simulink model "k1vistmsy"  (Simulink 8.6)
settings: Solver=ode45  StartTime=0.0  StopTime=10.0  RelTol=1e-3
libraries: VIS_TMS_LIB x3, cdsCDI64 x2, cdsCDO64 x2, cdsIPCx x2, cdsAdcx0 x1, cdsAdcx1 x1, cdsAdcx2 x1, dac x1, simulink x1, cdsParameters x1
settings Model: Creator=controls  LastModifiedBy=controls
settings OptimizationCC: InitFltsAndDblsToZero=on
settings DebuggingCC: FcnCallInpInsideContextMsg=EnableAllAsWarning  AllowSymbolicDim=on  StrictBusMsg=Warning

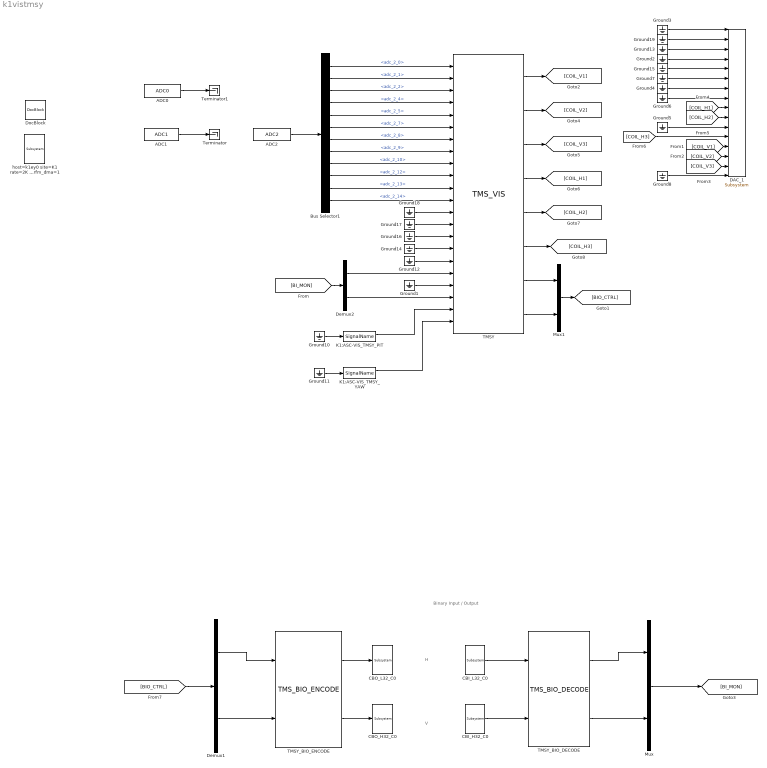
== system k1vistmsy ==
  note: Binary Input / Output
  note: H
  note: V
  ADC0 : cdsAdcx0/ADC0  Tag=cdsAdc  Description=|
      | type-GSC_16AI64SSA
      | card_num=0
      settings: AttributesFormatString=%<Description>\n%<Tag>
  ADC1 : cdsAdcx1/ADC1  Tag=cdsAdc  Description=|
      | type-GSC_16AI64SSA
      | card_num=1
      settings: AttributesFormatString=%<Description>\n%<Tag>
  ADC2 : cdsAdcx2/ADC2  Tag=cdsAdc  Description=|
      | type-GSC_16AI64SSA
      | card_num=2
      settings: AttributesFormatString=%<Description>\n%<Tag>
  Bus Selector1 : BusSelector  Description=ADC Selector  OutputSignals=adc_2_0,adc_2_1,adc_2_2,adc_2_4,adc_2_5,adc_2_7,adc_2_8,adc_2_9,adc_2_10,adc_2_12,adc_2_13,adc_2_14
      settings: AttributesFormatString=%<Description>
  CBI_H32_C0 : cdsCDI64/Subsystem  Tag=cdsCDI64  Description=card_num=1
      settings: AttributesFormatString=%<Tag>\n%<Description>
  CBI_L32_C0 : cdsCDI64/Subsystem  Tag=cdsCDI64  Description=card_num=0
      settings: AttributesFormatString=%<Tag>\n%<Description>
  CBO_H32_C0 : cdsCDO64/Subsystem  Tag=cdsCDO64  Description=card_num=1
      settings: AttributesFormatString=%<Tag>\n%<Description>
  CBO_L32_C0 : cdsCDO64/Subsystem  Tag=cdsCDO64  Description=card_num=0
      settings: AttributesFormatString=%<Tag>\n%<Description>
  DAC_1 : dac/Subsystem  Description=|
      | type=GSC_16AO16,
      | card_num=1
      settings: AttributesFormatString=%<Description>
  Demux1 : Demux  Outputs=2
  Demux2 : Demux  Outputs=2
  DocBlock : simulink/Model-Wide Utilities/DocBlock  DocumentType=Text
  Ground{1..8,10..19} (18 alike) : Ground
  K1:ASC-VIS_TMSY_PIT : cdsIPCx/SignalName  Tag=cdsIPCx_RFM  Description=card=1
      settings: AttributesFormatString=%<Description>\n%<Tag>
  K1:ASC-VIS_TMSY_YAW : cdsIPCx/SignalName  Tag=cdsIPCx_RFM  Description=card=1
      settings: AttributesFormatString=%<Description>\n%<Tag>
  Mux : Mux  Inputs=2
  Mux1 : Mux  Inputs=2
  TMSY : VIS_TMS_LIB/TMS_VIS
  TMSY_BIO_DECODE : VIS_TMS_LIB/TMS_BIO_DECODE
  TMSY_BIO_ENCODE : VIS_TMS_LIB/TMS_BIO_ENCODE
  Terminator : Terminator
  Terminator1 : Terminator
  host=k1ey0 site=K1 rate=2K dcuid=114 specific_cpu=6 adcSlave=1 no_rfm_dma=1 : cdsParameters/Subsystem  Tag=cdsParameters  Description=|
      | Purpose:                                                                                                                                                                                                                                
      |                                                                                                                                                                                                                                         
      | Provide system parameters to the FE code generator to properly configure the generated EPICS names, rep rate of the FE controller, and the Data Acquisition node ID for proper storage of data from this FE controller.                 
      |                                                                                                                                                                                                                                         
      | Useage:                                                                                                                                                                                                                                 
      |                                                                                                                                                                                                                                         
      | The part NAME field is used to identify the FE parameters. It must be of the form:                                                                                                                                                      
      |                                                                                                                                                                                                                                         
      | site=                                                                                                                                                                                                                                   
      | rate=                                                                                                                                                                                                                                   
      | dcuid=                                                                                                                                                                                                                                  
      |                                                                                                                                                                                                                                         
      | Where:                                                                                                                                                                                                                                  
      |                                                                                                                                                                                                                                         
      | site= argument may be H1, H2, L1, M1, G1, either as a single argument or multiple, for example site=H1,H2. These are the only names allowed. These will become the first two characters of all EPICS and signal names (for example G1:).
      |                                                                                                                                                                                                                                         
      | rate= may be 2K, 16K, 32K, or 64K                                                                                                                                                                                                       
      |                                                                                                                                                                                                                                         
      | dcuid= is site specific ie it must be unique at each site.
      settings: AttributesFormatString=%<Tag>
  wires:
  Bus Selector1/10 -> TMSY/10  "<adc_2_12>"
  Bus Selector1/11 -> TMSY/11  "<adc_2_13>"
  Bus Selector1/12 -> TMSY/12  "<adc_2_14>"
  TMSY_BIO_ENCODE/1 -> CBO_L32_C0/1
  CBI_L32_C0/1 -> TMSY_BIO_DECODE/1
  TMSY_BIO_DECODE/2 -> Mux/2
  TMSY_BIO_DECODE/1 -> Mux/1
  Mux/1 -> [BI_MON]
  [BIO_CTRL] -> Demux1/1
  TMSY_BIO_ENCODE/2 -> CBO_H32_C0/1
  Demux1/1 -> TMSY_BIO_ENCODE/1
  Demux1/2 -> TMSY_BIO_ENCODE/2
  CBI_H32_C0/1 -> TMSY_BIO_DECODE/2
  [BI_MON] -> Demux2/1
  TMSY/7 -> Mux1/1
  TMSY/8 -> Mux1/2
  Mux1/1 -> [BIO_CTRL]
  Demux2/1 -> TMSY/18
  Ground1/1 -> TMSY/19
  Ground12/1 -> TMSY/17
  Demux2/2 -> TMSY/20
  Bus Selector1/1 -> TMSY/1  "<adc_2_0>"
  Bus Selector1/2 -> TMSY/2  "<adc_2_1>"
  Bus Selector1/3 -> TMSY/3  "<adc_2_2>"
  Bus Selector1/4 -> TMSY/4  "<adc_2_4>"
  Bus Selector1/5 -> TMSY/5  "<adc_2_5>"
  Bus Selector1/6 -> TMSY/6  "<adc_2_7>"
  Bus Selector1/7 -> TMSY/7  "<adc_2_8>"
  Bus Selector1/8 -> TMSY/8  "<adc_2_9>"
  Bus Selector1/9 -> TMSY/9  "<adc_2_10>"
  Ground10/1 -> K1:ASC-VIS_TMSY_PIT/1
  Ground11/1 -> K1:ASC-VIS_TMSY_YAW/1
  K1:ASC-VIS_TMSY_PIT/1 -> TMSY/21
  K1:ASC-VIS_TMSY_YAW/1 -> TMSY/22
  ADC2/1 -> Bus Selector1/1
  Ground14/1 -> TMSY/16
  Ground16/1 -> TMSY/15
  Ground17/1 -> TMSY/14
  Ground18/1 -> TMSY/13
  Ground15/1 -> DAC_1/5
  Ground3/1 -> DAC_1/1
  Ground13/1 -> DAC_1/3
  Ground2/1 -> DAC_1/4
  TMSY/1 -> [COIL_V1]
  TMSY/2 -> [COIL_V2]
  TMSY/6 -> [COIL_H3]
  TMSY/5 -> [COIL_H2]
  TMSY/4 -> [COIL_H1]
  TMSY/3 -> [COIL_V3]
  Ground7/1 -> DAC_1/6
  Ground4/1 -> DAC_1/7
  Ground6/1 -> DAC_1/8
  Ground8/1 -> DAC_1/16
  [COIL_V1] -> DAC_1/13
  [COIL_V2] -> DAC_1/14
  [COIL_V3] -> DAC_1/15
  ADC1/1 -> Terminator/1
  ADC0/1 -> Terminator1/1
  [COIL_H1] -> DAC_1/9
  [COIL_H2] -> DAC_1/10
  Ground19/1 -> DAC_1/2
  Ground5/1 -> DAC_1/11
  [COIL_H3] -> DAC_1/12
